simulink model "AAI"  (R2020a)
settings: Solver=FixedStepAuto  StartTime=0.0  StopTime=10.0  FixedStep=1e-3  RelTol=1e-3  EnableMultiTasking=on
undefined symbols (not defined in the file): D0, D10, D11, D12, D13, D2, D4, D5, D6, D7, D8, D9, PTA0, PTA2, PTB23, PTB9, PTC16, PTC2, PTC3, PTC4, PTD0, PTD1, PTD2, PTD3
libraries: frdmk64flib x12
settings Model: ExtModeTrigDuration=5  Creator=Abrar Hussain  LastModifiedBy=Nabil
settings OptimizationCC: EnhancedBackFolding=on  PassReuseOutputArgsAs=Individual arguments  ZeroExternalMemoryAtStartup=off  ZeroInternalMemoryAtStartup=off  MaxStackSize=64  OptimizeBlockOrder=speed  DifferentSizesBufferReuse=on  OptimizationCustomize=off  EfficientTunableParamExpr=on
settings DebuggingCC: ParameterTunabilityLossMsg=error
settings HardwareCC: ProdBitPerPointer=32  ProdBitPerSizeT=32  ProdBitPerPtrDiffT=32  ProdLargestAtomicInteger=Long  ProdLargestAtomicFloat=Double  ProdWordSize=32  ProdHWDeviceType=ARM Compatible->ARM Cortex
settings SFSimCC: MATLABDynamicMemAlloc=off
settings RTWCC: SystemTargetFile=ert.tlc  HardwareBoard=NXP FRDM-K64F  TemplateMakefile=ert_default_tmf  Toolchain=GNU Tools for ARM Embedded Processors
settings CodeAppCC: ForceParamTrailComments=on  IgnoreCustomStorageClasses=off  OperatorAnnotations=on  SimulinkDataObjDesc=on  SFDataObjDesc=on  InsertBlockDesc=on

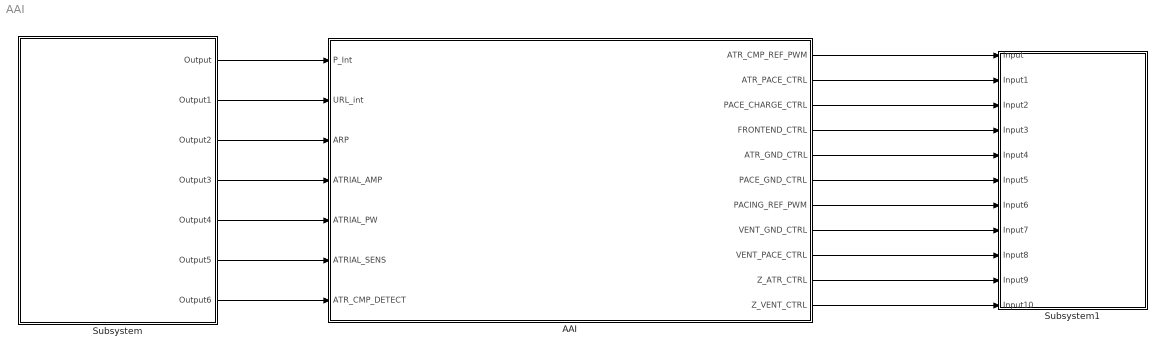
== system AAI ==
  AAI : Stateflow chart  TreatAsAtomicUnit=on
  Subsystem : Subsystem
  Subsystem1 : Subsystem
  wires:
  Subsystem/1(Output) -> AAI/1(P_Int)
  Subsystem/2(Output1) -> AAI/2(URL_int)
  Subsystem/3(Output2) -> AAI/3(ARP)
  Subsystem/4(Output3) -> AAI/4(ATRIAL_AMP)
  Subsystem/5(Output4) -> AAI/5(ATRIAL_PW)
  Subsystem/6(Output5) -> AAI/6(ATRIAL_SENS)
  Subsystem/7(Output6) -> AAI/7(ATR_CMP_DETECT)
  AAI/1(ATR_CMP_REF_PWM) -> Subsystem1/1(Input)
  AAI/2(ATR_PACE_CTRL) -> Subsystem1/2(Input1)
  AAI/3(PACE_CHARGE_CTRL) -> Subsystem1/3(Input2)
  AAI/4(FRONTEND_CTRL) -> Subsystem1/4(Input3)
  AAI/5(ATR_GND_CTRL) -> Subsystem1/5(Input4)
  AAI/6(PACE_GND_CTRL) -> Subsystem1/6(Input5)
  AAI/7(PACING_REF_PWM) -> Subsystem1/7(Input6)
  AAI/8(VENT_GND_CTRL) -> Subsystem1/8(Input7)
  AAI/9(VENT_PACE_CTRL) -> Subsystem1/9(Input8)
  AAI/10(Z_ATR_CTRL) -> Subsystem1/10(Input9)
  AAI/11(Z_VENT_CTRL) -> Subsystem1/11(Input10)

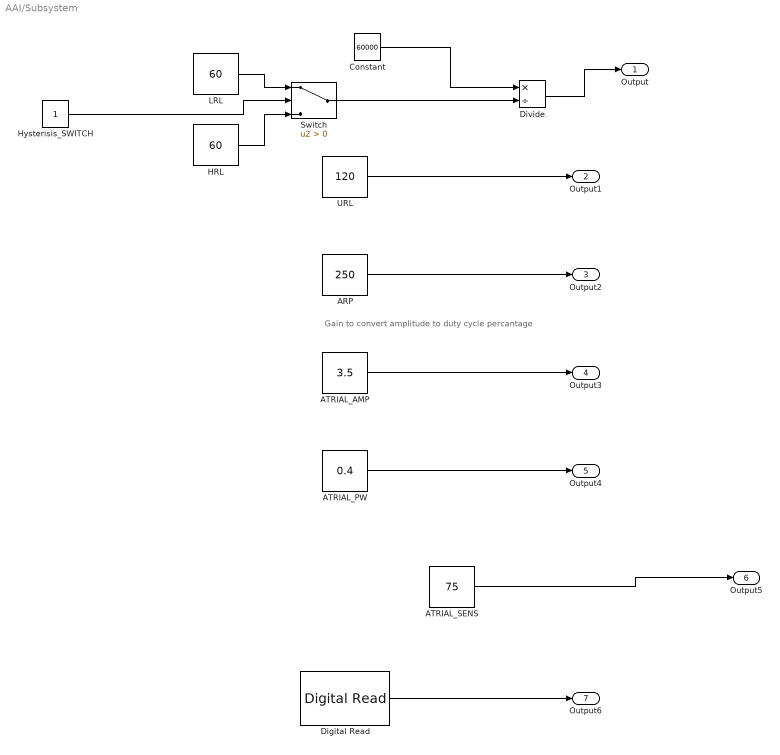
== system AAI/Subsystem ==
  note: Gain to convert amplitude to duty cycle percantage
  ARP : Constant  Value=250
  ATRIAL_AMP : Constant  Value=3.5
  ATRIAL_PW : Constant  Value=0.4
  ATRIAL_SENS : Constant  Value=75
  Constant : Constant  Value=60000
  Digital Read : frdmk64flib/Digital Read  Whichpin=PTC16 (D0)  SampleTime=-1
  Divide : Product  Inputs=*/
  HRL : Constant  Value=60
  Hysterisis_SWITCH : Constant
  LRL : Constant  Value=60
  Switch : Switch  Criteria=u2 > Threshold
  URL : Constant  Value=120
  Output : Outport
  Output1 : Outport  Port=2
  Output2 : Outport  Port=3
  Output3 : Outport  Port=4
  Output4 : Outport  Port=5
  Output5 : Outport  Port=6
  Output6 : Outport  Port=7
  wires:
  URL/1 -> Output1/1
  ARP/1 -> Output2/1
  Digital Read/1 -> Output6/1
  ATRIAL_AMP/1 -> Output3/1
  ATRIAL_PW/1 -> Output4/1
  ATRIAL_SENS/1 -> Output5/1
  Constant/1 -> Divide/1
  Divide/1 -> Output/1
  HRL/1 -> Switch/3
  Hysterisis_SWITCH/1 -> Switch/2
  Switch/1 -> Divide/2
  LRL/1 -> Switch/1

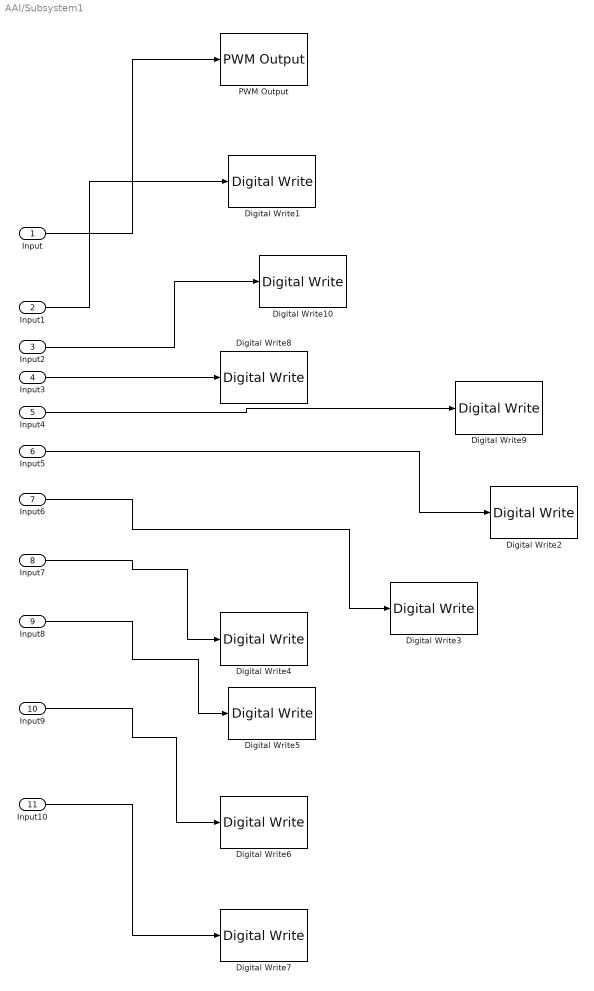
== system AAI/Subsystem1 ==
  Input : Inport
  Input1 : Inport  Port=2
  Input2 : Inport  Port=3
  Input3 : Inport  Port=4
  Input4 : Inport  Port=5
  Input5 : Inport  Port=6
  Input6 : Inport  Port=7
  Input7 : Inport  Port=8
  Input8 : Inport  Port=9
  Input9 : Inport  Port=10
  Input10 : Inport  Port=11
  Digital Write1 : frdmk64flib/Digital Write  Whichpin=PTA0 (D8)
  Digital Write10 : frdmk64flib/Digital Write  Whichpin=PTB9 (D2)
  Digital Write2 : frdmk64flib/Digital Write  Whichpin=PTD0 (D10)
  Digital Write3 : frdmk64flib/Digital Write  Whichpin=PTA2 (D5)
  Digital Write4 : frdmk64flib/Digital Write  Whichpin=PTD3 (D12)
  Digital Write5 : frdmk64flib/Digital Write  Whichpin=PTC4 (D9)
  Digital Write6 : frdmk64flib/Digital Write  Whichpin=PTB23 (D4)
  Digital Write7 : frdmk64flib/Digital Write  Whichpin=PTC3 (D7)
  Digital Write8 : frdmk64flib/Digital Write  Whichpin=PTD1 (D13)
  Digital Write9 : frdmk64flib/Digital Write  Whichpin=PTD2 (D11)
  PWM Output : frdmk64flib/PWM Output  Whichpin=PTC2 (D6)  InitialFrequency=2000  InitialDutyCycle=0
  wires:
  Input/1 -> PWM Output/1
  Input1/1 -> Digital Write1/1
  Input10/1 -> Digital Write7/1
  Input9/1 -> Digital Write6/1
  Input8/1 -> Digital Write5/1
  Input7/1 -> Digital Write4/1
  Input6/1 -> Digital Write3/1
  Input5/1 -> Digital Write2/1
  Input4/1 -> Digital Write9/1
  Input3/1 -> Digital Write8/1
  Input2/1 -> Digital Write10/1

== stateflow chart AAI/AAI ==
  state Pacing
    entry:
    %sensing off
    FRONTEND_CTRL = 0;
    %PACE
    PACE_CHARGE_CTRL = 0;
    PACE_GND_CTRL = 1;
    VENT_PACE_CTRL = 0;
    VENT_GND_CTRL = 0;
    Z_VENT_CTRL = 0;
    Z_ATR_CTRL = 0;
    ATR_GND_CTRL = 0;
    ATR_PACE_CTRL = 1;
    PACING_REF_PWM = ATRIAL_AMP;
  state C22_Charge_C21_Discharge
    entry:
    FRONTEND_CTRL = 1; %sensing ON
    %C22 Charge
    VENT_PACE_CTRL = 0;
    ATR_PACE_CTRL = 0;
    PACING_REF_PWM = ATRIAL_AMP;
    PACE_CHARGE_CTRL = 1;
    %We can also discharge C21 from previous pacing
    PACE_GND_CTRL = 1;
    ATR_PACE_CTRL = 0;
    Z_VENT_CTRL = 0;
    Z_ATR_CTRL = 0;
    VENT_PACE_CTRL = 0;
    VENT_GND_CTRL = 0;
    ATR_GND_CTRL = 1;
    ATR_CMP_REF_PWM = ATRIAL_SENS;
  state ARP_Period
    entry:
    FRONTEND_CTRL = 0; % No sensing
    ATR_PACE_CTRL = 0;
    VENT_PACE_CTRL = 0;
    %ATR_GND_CTRL = 1;
    %PACE_CHARGE_CTRL = 0;
    %PACE_GND_CTRL = 1;
    PACING_REF_PWM = ATRIAL_AMP
  (default) -> C22_Charge_C21_Discharge
  C22_Charge_C21_Discharge -> (junction 58)
  (junction 58) -> Pacing [order 1] : [(ATR_CMP_DETECT == false ) && after(P_Int - ATRIAL_PW - ARP,msec)]
  (junction 58) -> ARP_Period [order 2] : [ATR_CMP_DETECT == true]
  ARP_Period -> C22_Charge_C21_Discharge : after(ARP,msec)
  Pacing -> ARP_Period : after(ATRIAL_PW, msec)
  data: P_Int input; URL_int input; ARP input; ATRIAL_AMP input; ATRIAL_PW input; ATRIAL_SENS input; ATR_CMP_DETECT input; ATR_CMP_REF_PWM output; ATR_PACE_CTRL output; PACE_CHARGE_CTRL output; FRONTEND_CTRL output; ATR_GND_CTRL output; PACE_GND_CTRL output; PACING_REF_PWM output; VENT_GND_CTRL output; VENT_PACE_CTRL output; Z_ATR_CTRL output; Z_VENT_CTRL output
